simulink model "PiekarekLab5_si"  (R2022b)
settings: Solver=VariableStepAuto  StartTime=0.0  StopTime=10.0  MaxStep=1  RelTol=1e-3
values from neighbouring files (symbols this model uses):
  dU = 5    [PiekarekLab5.m]
  Kp1 = 1.5*((0.9*T)/(k*T0))    (= 3150)    [PiekarekLab5.m]
  L = [k]    [PiekarekLab5.m]
  M = [140,1]    [PiekarekLab5.m]
  T0 = 20    [PiekarekLab5.m]
  Ti = 3.33*T0    (= 66.6)    [PiekarekLab5.m]
settings Model: Creator=Lenovo  LastModifiedBy=Lenovo

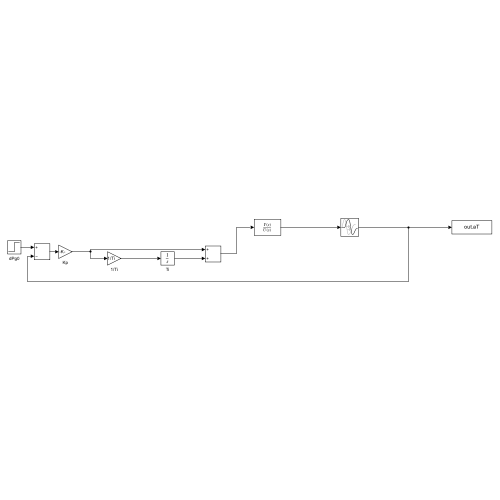
[thumbnail: Simulink's stored preview of the top-level diagram]
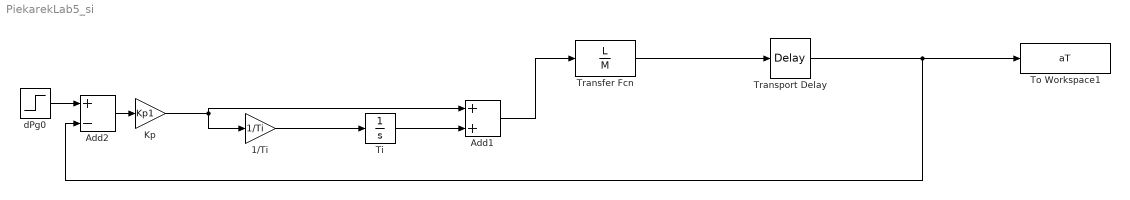
== system PiekarekLab5_si ==
  1/Ti : Gain  Gain=1/Ti
  Add1 : Sum
  Add2 : Sum  Inputs=+-
  Kp : Gain  Gain=Kp1
  Ti : Integrator  InitialCondition=Ti
  To Workspace1 : ToWorkspace  VariableName=aT  SampleTime=-1
  Transfer Fcn : TransferFcn  Numerator=L  Denominator=M
  Transport Delay : TransportDelay  DelayTime=T0
  dPg0 : Step  Time=0  After=dU  SampleTime=0
  wires:
  Transport Delay/1 -> Add2/2, To Workspace1/1
  Transfer Fcn/1 -> Transport Delay/1
  Add1/1 -> Transfer Fcn/1
  Ti/1 -> Add1/2
  1/Ti/1 -> Ti/1
  Kp/1 -> 1/Ti/1, Add1/1
  dPg0/1 -> Add2/1
  Add2/1 -> Kp/1
